simulink model "Driver_testing"  (R2019b)
settings: Solver=VariableStepAuto  StartTime=0.0  StopTime=10  MaxStep=0.01  RelTol=1e-3
InitFcn:
  | F_Rider = 85;
  | Brake_Pressure = 0;
  | Crank_Length = 0.150;
  | Angle_of_crank = [0:1:360;0:1:360;]';
settings Model: Creator=Avmash  LastModifiedBy=Avmash

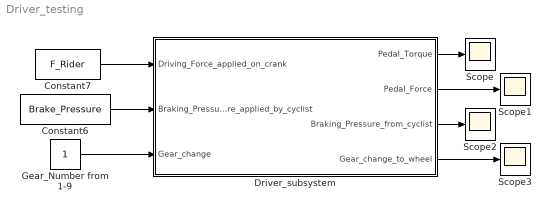
== system Driver_testing ==
  Constant6 : Constant  Value=Brake_Pressure
  Constant7 : Constant  Value=F_Rider
  Driver_subsystem : Subsystem
  Gear_Number from 1-9 : Constant
  Scope{,1..3} (4 alike) : Scope
  wires:
  Gear_Number from 1-9/1 -> Driver_subsystem/3(Gear_change)
  Constant6/1 -> Driver_subsystem/2(Braking_Pressure_applied_by_cyclist)
  Constant7/1 -> Driver_subsystem/1(Driving_Force_applied_on_crank)
  Driver_subsystem/1(Pedal_Torque) -> Scope/1
  Driver_subsystem/2(Pedal_Force) -> Scope1/1
  Driver_subsystem/3(Braking_Pressure_from_cyclist) -> Scope2/1
  Driver_subsystem/4(Gear_change_to_wheel) -> Scope3/1

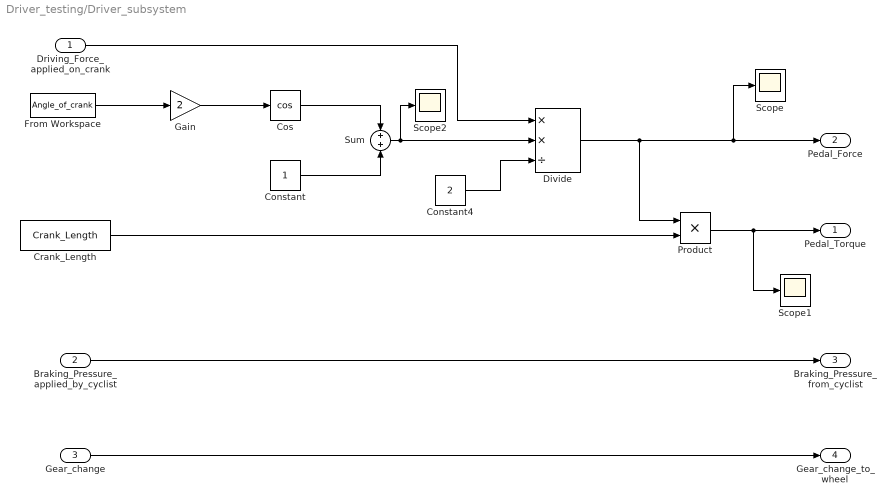
== system Driver_testing/Driver_subsystem ==
  Driving_Force_applied_on_crank : Inport
  Braking_Pressure_applied_by_cyclist : Inport  Port=2
  Gear_change : Inport  Port=3
  Constant : Constant
  Constant4 : Constant  Value=2
  Cos : Trigonometry  Operator=cos
  Crank_Length : Constant  Value=Crank_Length
  Divide : Product  Inputs=**/
  From Workspace : FromWorkspace  VariableName=Angle_of_crank  SampleTime=0
  Gain : Gain  Gain=2
  Product : Product
  Scope : Scope
  Scope1 : Scope
  Scope2 : Scope
  Sum : Sum
  Pedal_Torque : Outport
  Pedal_Force : Outport  Port=2
  Braking_Pressure_from_cyclist : Outport  Port=3
  Gear_change_to_wheel : Outport  Port=4  VectorParamsAs1DForOutWhenUnconnected=off
  wires:
  Divide/1 -> Scope/1, Pedal_Force/1, Product/1
  Gain/1 -> Cos/1
  Constant/1 -> Sum/2
  Cos/1 -> Sum/1
  Product/1 -> Scope1/1, Pedal_Torque/1
  Constant4/1 -> Divide/3
  Driving_Force_applied_on_crank/1 -> Divide/1
  Sum/1 -> Scope2/1, Divide/2
  Crank_Length/1 -> Product/2
  Braking_Pressure_applied_by_cyclist/1 -> Braking_Pressure_from_cyclist/1
  From Workspace/1 -> Gain/1
  Gear_change/1 -> Gear_change_to_wheel/1
